simulink model "labA23"  (R2025b)
settings: Solver=ode45  StartTime=0.0  StopTime=300  RelTol=1e-3  AbsTol=1e-3  EnableMultiTasking=on
StopFcn:
  | %% Colors
  | 
  | blue = [0, 0.4470, 0.7410]; % RGB for blue
  | red = [0.8500, 0.3250, 0.0980]; % RGB for red
  | green = [0, 0.4980, 0]; % RGB for green
  | 
  | %% Data fetching
  | rt    = simout.u_v1.time; s.t=rt;  % time vector
  | ru_v1 = simout.u_v1.data; s.u_v1=ru_v1;
  | ru_v2 = simout.u_v2.data; s.u_v2=ru_v1;
  | ru_p  = simout.u_p.data;  s.u_p=ru_p;
  | rh1   = simout.measurement1.data; s.h1=rh1;
  | rh1_ref = simout.model1.data; s.h1_ref=rh1_ref;
  | rh2   = simout.measurement2.data; s.h2=rh2;
  | rh2_ref = simout.model2.data; s.h2_ref=rh2_ref;
  | 
  | %% Create figure
  | rslt = figure('Name','Results','Units','normalized', ...
  |               'Position',[0.25 0.2 0.5 0.5], ...
  |               'Color','w');
  | 
  | % Create tiled layout (3x2)
  | tl = tiledlayout(3,2,'Padding','compact','TileSpacing','compact');
  | 
  | %% Tile 1: u_v1
  | nexttile
  | plot(rt, ru_v1, 'Color', blue, 'LineWidth', 1.5)
  | xlabel('Time [s]')
  | ylabel('Valve signal u_{v1} [-]')
  | grid on;
  | 
  | %% Tile 2: h1
  | nexttile
  | plot(rt, rh1, 'Color', blue, 'LineWidth', 1.5)
  | hold on;
  | plot(rt, rh1_ref, 'Color', red, 'LineWidth', 1.5)
  | xlabel('Time [s]'); ylabel('Height h1 [m]'); grid on;
  | 
  | %% Tile 3: u_v2
  | nexttile
  | plot(rt, ru_v2, 'Color', blue, 'LineWidth', 1.5)
  | xlabel('Time [s]')
  | ylabel('Valve signal u_{v2} [-]')
  | grid on;
  | 
  | %% Tile 4: h2
  | nexttile
  | plot(rt, rh2, 'Color', blue, 'LineWidth', 1.5)
  | hold on;
  | plot(rt, rh2_ref, 'Color', red, 'LineWidth', 1.5)
  | xlabel('Time [s]'); ylabel('Height h2 [m]'); grid on;
  | 
  | %% Tile 5: u_p
  | nexttile
  | plot(rt, ru_p, 'Color', blue, 'LineWidth', 1.5)
  | xlabel('Time [s]')
  | ylabel('Pump signal u_{p} [-]')
  | grid on;
  | 
  | sgtitle('Results', 'FontWeight','bold');
undefined symbols (not defined in the file or in its folder): A1, f_v1, f_v2, g, h1_max, h1_min, h2_max, h2_min, h_v1, h_v2, k_v1, k_v2, q_p, rho, u_p, u_v1, u_v2, X, Y, Z
libraries: sm_lib x21, nesl_utility x8
settings Model: PacingRate=8  Creator=2922887  LastModifiedBy=danie
settings SolverCC: AutoScaleAbsTol=off  AlgebraicLoopSolver=TrustRegion
settings DataIOCC: LimitDataPoints=on  MaxDataPoints=10000  ReturnWorkspaceOutputs=off
settings OptimizationCC: LifeSpan=inf
settings DebuggingCC: UnconnectedInputMsg=warning  UnconnectedOutputMsg=warning  UnconnectedLineMsg=warning  AllowSymbolicDim=off  SFUnexpectedBacktrackingDiag=warning  SFNoUnconditionalDefaultTransitionDiag=warning  SFExecutionAtInitializationDiag=none  ArithmeticOperatorsInVariantConditions=warning
settings ModelReferenceCC: EnableRefExpFcnMdlSchedulingChecks=on
settings SFSimCC: SimUseLocalCustomCode=off  CustomCodeUndefinedFunction=UseInterfaceOnly
settings RTWCC: RTWUseLocalCustomCode=off  GPUComputeCapability=3.5  DLArmComputeVersion=19.05
settings CodeAppCC: StateflowObjectComments=on
settings GRTTargetCC: TargetLangStandard=C89/C90 (ANSI)
settings ConfigComp: CovMetricSettings=dw  CovSaveCumulativeToWorkspaceVar=on  CovSaveSingleToWorkspaceVar=on  CovExternalEMLEnable=off  CovSFcnEnable=off
settings SimscapeCC: SimscapeLogType=all  SimscapeLogSimulationStatistics=on  SimscapeLogDataHistory=10000.0
settings ExplorerConfigSet: InternalSimMechanicsExplorerSettings="<ExplorerConfiguration><canonicalview>default</canonicalview><AnimationSetting><BasePlaybackSpeed>1.0</BasePlaybackSpeed><PlaybackSpeedFactor>256.0</PlaybackSpeedFactor></AnimationSetting><TilePanel><TileInfo><Tiles Columns=\"1\" Count=\"1\" Rows=\"1\"><Column Weight=\"1\"/><Row Weight=\"1\"/><Tile Height=\"1\" Width=\"1\" X=\"0\" Y=\"0\"/></Tiles></TileInfo><SceneInfo><SceneViewer><BGColor><R>1</R><G>1</G><B>1</B></BGColor><Camera><DoPerspective>off</DoPerspective><Position><X>1.74662213976138903</X><Y>-0.732674940485340098</Y><Z>1.86695078489503663</Z></Position><Center><X>-0.869514407391283939</X><Y>0.382598842481733703</Y><Z>0.955734133281551657</Z></Center><Up><X>-0.285163512035032929</X><Y>0.109102028578263566</Y><Z>0.952249189426777054</Z></Up><ViewLimDist>1</ViewLimDist><YLim>1.42715679542026352</YLim><XLim>2.09465770497110215</XLim></Camera></SceneViewer></SceneInfo></TilePanel><MechEditorPanel><Cameras/><GfxPanelCameraMap/><VideoCreator><PlaybackSpeedRatio>1.0</PlaybackSpeedRatio><FrameRate>30</FrameRate><VideoFormat>Motion JPEG AVI</VideoFormat><FrameSize>auto</FrameSize></VideoCreator></MechEditorPanel></ExplorerConfiguration>"

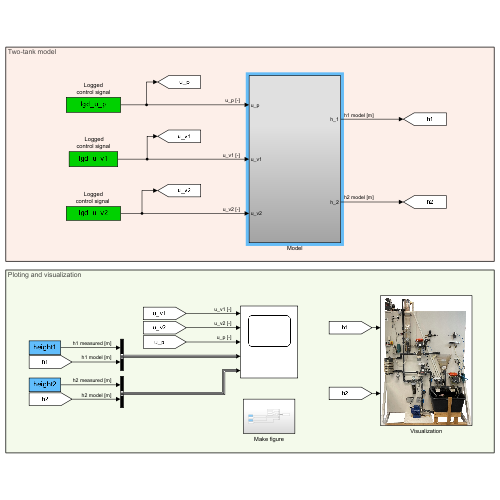
[thumbnail: Simulink's stored preview of the top-level diagram]
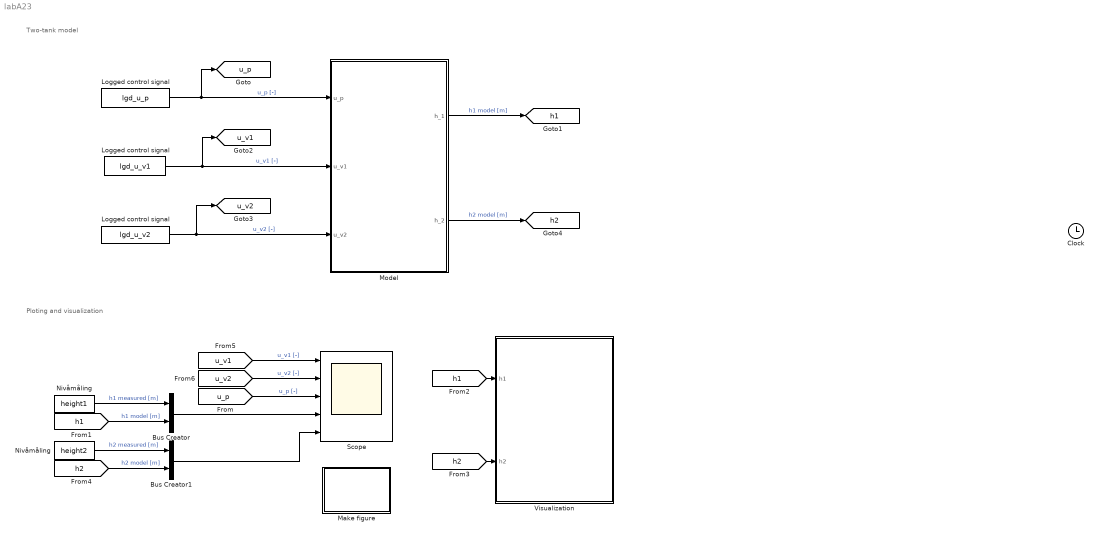
== system labA23 ==
  note: Ploting and visualization
  note: Two-tank model
  " Logged control signal" : FromWorkspace  VariableName=lgd_u_v1  SampleTime=0.07
  Bus Creator : BusCreator  Inputs=2
  Bus Creator1 : BusCreator  Inputs=2
  Logged control signal : FromWorkspace  VariableName=lgd_u_p  SampleTime=0.07
  "Logged control signal " : FromWorkspace  VariableName=lgd_u_v2  SampleTime=0.07
  Make figure : Subsystem
  Model : Subsystem
  Nivåmåling : FromWorkspace  VariableName=height1  SampleTime=0.07
  "Nivåmåling " : FromWorkspace  VariableName=height2  SampleTime=0.07
  Scope : Scope  NumInputPorts=5
      settings: TimeSpan=300  ActiveDisplayYMinimum=-0.125  ActiveDisplayYMaximum=1.125
  Visualization : Subsystem  mask{visualization=Visualization off, PacingRate=8}
      mask prompts: PacingRate "Simulation ratio (1:x) time vs real time"
      settings: PortSchema="{\"entries\":[{\"content\":{\"sides\":[{\"content\":{\"connectorIds\":[]},\"type\":\"ConnectorPlacement.EquallySpacedRectSide\",\"uuid\":\"ef884aaa-3eab-45c5-b5e8-52d600c009e8\"},{\"content\":{\"connectorIds\":[\"In1\",\"In2\"],\"side\":\"RIGHT\"},\"type\":\"ConnectorPlacement.EquallySpacedRectSide\",\"uuid\":\"bd48a19f-380a-480a-b360-7685a60cdefc\"},{\"content\":{\"connectorIds\":[],\"side\":\"TOP\"},\"type\":\"ConnectorPlacement.EquallySpacedRectSide\",\"uuid\":\"e0bb9c54-6b8d-425a-9dcd-efa9c2145964\"},{\"content\":{\"connectorIds\":[],\"side\":\"HIDDEN\"},\"type\":\"ConnectorPlacement.EquallySpacedRectSide\",\"uuid\":\"043d02d6-7b77-4bef-801d-231041ca0e56\"}]},\"type\":\"ConnectorPlacement.EquallySpacedConnector\",\"uuid\":\"8c6c52bd-5deb-48d7-b067-5e5f394c76bc\"}],\"packageUris\":[\"http://schema.mathworks.com/mf0/Connector/R2020b\"],\"version\":\"1.0\"}"
      mask TypeOptions visualization: Visualization  on | Visualization off
      mask Callback visualization:
      | if get_param(append(bdroot,'/Visualization'),'visualization') == 'Visualization  on'
      |    set_param(bdroot,'EnablePacing','on')
      | elseif get_param(append(bdroot,'/Visualization'),'visualization') == 'Visualization off'
      |    set_param(bdroot,'EnablePacing','off')
      | end
      mask Callback PacingRate:
      | temp_param = str2num(get_param(append(bdroot,'/Visualization'),'PacingRate'));
      | if temp_param >= 0.003 && temp_param < 0.0078
      |     set_param(bdroot,'PacingRate','0.0039')
      |     set_param(append(bdroot,'/Visualization'),'PacingRate','0.0039')
      | elseif temp_param >= 0.0078 && temp_param < 0.0156
      |     set_param(bdroot,'PacingRate','0.0078')
      |     set_param(append(bdroot,'/Visualization'),'PacingRate','0.0078')
      | elseif temp_param >= 0.0156 && temp_param < 0.0313
      |     set_param(bdroot,'PacingRate','0.0156')
      |     set_param(append(bdroot,'/Visualization'),'PacingRate','0.0156')
      | elseif temp_param >= 0.0313 && temp_param < 0.0625
      |     set_param(bdroot,'PacingRate','0.0313')
      |     set_param(append(bdroot,'/Visualization'),'PacingRate','0.0313')
      | elseif temp_param >= 0.0625 && temp_param < 0.1250
      |     set_param(bdroot,'PacingRate','0.0625')
      |     set_param(append(bdroot,'/Visualization'),'PacingRate','0.0625')
      | elseif temp_param >= 0.1250 && temp_param < 0.2500
      |     set_param(bdroot,'PacingRate','0.1250')
      |     set_param(append(bdroot,'/Visualization'),'PacingRate','0.1250')
      | elseif temp_param >= 0.2500 && temp_param < 0.5000
      |     set_param(bdroot, 'PacingRate','0.2500')
      |     set_param(append(bdroot,'/Visualization'),'PacingRate','0.2500')
      | elseif temp_param >= 0.5000 && temp_param < 1
      |     set_param(bdroot, 'PacingRate','0.5000')
      |     set_param(append(bdroot,'/Visualization'),'PacingRate','0.5000')
      | elseif temp_param >= 1 && temp_param < 2
      |     set_param(bdroot, 'PacingRate','1')
      |     set_param(append(bdroot,'/Visualization'),'PacingRate','1')
      | elseif temp_param >= 2 && temp_param < 4
      |     set_param(bdroot, 'PacingRate','2')
      |     set_param(append(bdroot,'/Visualization'),'PacingRate','2')
      | elseif temp_param >= 4 && temp_param < 8
      |     set_param(bdroot, 'PacingRate','4')
      |     set_param(append(bdroot,'/Visualization'),'PacingRate','4')
      | elseif temp_param >= 8 && temp_param < 16
      |     set_param(bdroot, 'PacingRate','8')
      |     set_param(append(bdroot,'/Visualization'),'PacingRate','8')
      | elseif temp_param >= 16 && temp_param < 32
      |     set_param(bdroot, 'PacingRate','16')
      |     set_param(append(bdroot,'/Visualization'),'PacingRate','16')
      | elseif temp_param >= 32 && temp_param < 64
      |     set_param(bdroot, 'PacingRate','32')
      |     set_param(append(bdroot,'/Visualization'),'PacingRate','32')
      | elseif temp_param >= 64 && temp_param < 128
      |     set_param(bdroot, 'PacingRate','64')
      |     set_param(append(bdroot,'/Visualization'),'PacingRate','64')
      | elseif temp_param >= 128 && temp_param < 256
      |     set_param(bdroot, 'PacingRate','128')
      |     set_param(append(bdroot,'/Visualisering'),'PacingRate','128')
      | elseif temp_param >= 256
      |     set_param(bdroot, 'PacingRate','256')
      |     set_param(append(bdroot,'/Visualization'),'PacingRate','256')
      | end
      mask DialogControl Control2 Prompt: For a 1:1 relation between the visualization model and the plotted data, the simulation ratio in this box should match the ratio in the Mechanics Explorer.
      mask DialogControl x256x Prompt: 0.0039 = 1/256x
      mask DialogControl x128x Prompt: 0.0078 = 1/128x
      mask DialogControl x64x Prompt: 0.0156 = 1/64x
      mask DialogControl x32x Prompt: 0.0313 = 1/32x
      mask DialogControl x16x Prompt: 0.0625 = 1/16x
      mask DialogControl x8x Prompt: 0.1250 = 1/8x
      mask DialogControl x4x Prompt: 0.2500 = 1/4x
      mask DialogControl x2x Prompt: 0.5000 = 1/2x
      mask Display: image('$imagefile'); % Use "Edit Image" on toolstrip to change.
  Clock : Clock
      settings: IOType=siggen
  tag scope: h1=global, h2=global, u_p=global, u_v1=global, u_v2=global
  wires:
  " Logged control signal"/1 -> [u_v1], Model/2(u_v1)  "u_v1 [-]"
  Model/1(h_1) -> [h1]  "h1 model [m]"
  Logged control signal/1 -> [u_p], Model/1(u_p)  "u_p [-]"
  Nivåmåling/1 -> Bus Creator/1  "h1 measured [m]"
  "Logged control signal "/1 -> [u_v2], Model/3(u_v2)  "u_v2 [-]"
  Model/2(h_2) -> [h2]  "h2 model [m]"
  [h1] -> Visualization/1(h1)
  [h2] -> Visualization/2(h2)
  [h1] -> Bus Creator/2  "h1 model [m]"
  [h2] -> Bus Creator1/2  "h2 model [m]"
  "Nivåmåling "/1 -> Bus Creator1/1  "h2 measured [m]"
  Bus Creator1/1 -> Scope/5
  Bus Creator/1 -> Scope/4
  [u_v2] -> Scope/2  "u_v2 [-]"
  [u_v1] -> Scope/1  "u_v1 [-]"
  [u_p] -> Scope/3  "u_p [-]"

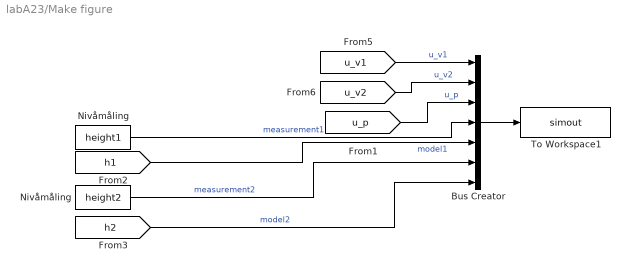
== system labA23/Make figure ==
  Bus Creator : BusCreator  Inputs=7
  Nivåmåling : FromWorkspace  VariableName=height1  SampleTime=0.07
  "Nivåmåling " : FromWorkspace  VariableName=height2  SampleTime=0.07
  To Workspace1 : ToWorkspace  VariableName=simout  SaveFormat=Timeseries  SampleTime=0.07
  wires:
  Bus Creator/1 -> To Workspace1/1
  [u_v1] -> Bus Creator/1  "u_v1"
  [u_v2] -> Bus Creator/2  "u_v2"
  [u_p] -> Bus Creator/3  "u_p"
  Nivåmåling/1 -> Bus Creator/4  "measurement1"
  [h1] -> Bus Creator/5  "model1"
  "Nivåmåling "/1 -> Bus Creator/6  "measurement2"
  [h2] -> Bus Creator/7  "model2"

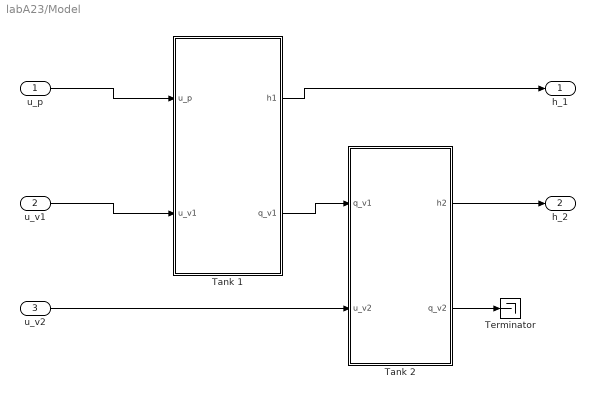
== system labA23/Model ==
  u_p : Inport
  u_v1 : Inport  Port=2
  u_v2 : Inport  Port=3
  Tank 1 : Subsystem
  Tank 2 : Subsystem
  Terminator : Terminator
  h_1 : Outport  VectorParamsAs1DForOutWhenUnconnected=off
  h_2 : Outport  Port=2  VectorParamsAs1DForOutWhenUnconnected=off
  wires:
  u_v1/1 -> Tank 1/2(u_v1)
  u_p/1 -> Tank 1/1(u_p)
  Tank 1/1(h1) -> h_1/1
  Tank 1/2(q_v1) -> Tank 2/1(q_v1)
  Tank 2/1(h2) -> h_2/1
  u_v2/1 -> Tank 2/2(u_v2)
  Tank 2/2(q_v2) -> Terminator/1

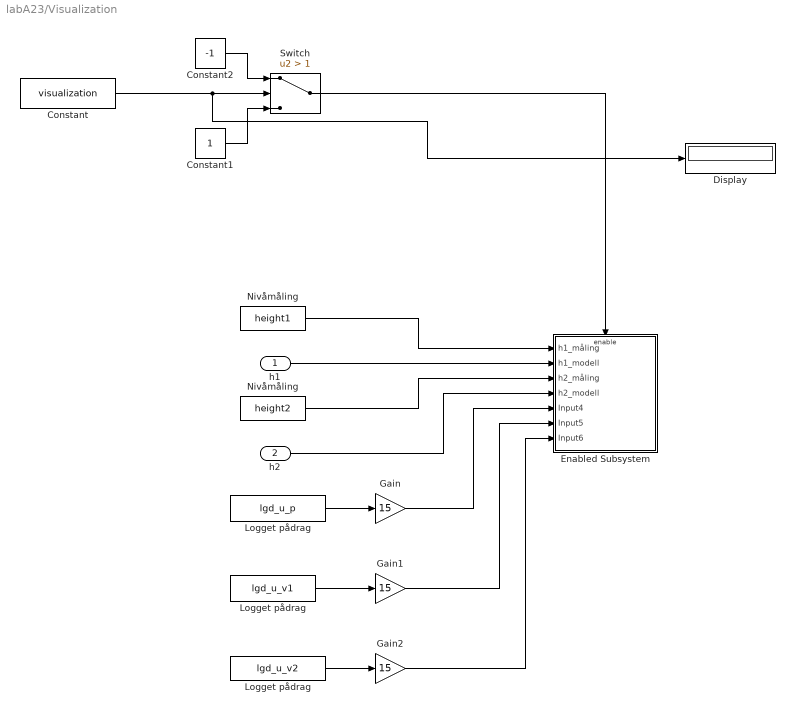
== system labA23/Visualization ==
  h1 : Inport
  h2 : Inport  Port=2
  Constant : Constant  Value=visualization
  Constant1 : Constant
  Constant2 : Constant  Value=-1
  Display : Display
  Enabled Subsystem : Subsystem  TreatAsAtomicUnit=on
  Gain : Gain  Gain=15
  Gain1 : Gain  Gain=15
  Gain2 : Gain  Gain=15
  Logget pådrag : FromWorkspace  VariableName=lgd_u_p  SampleTime=0.07
  "Logget pådrag " : FromWorkspace  VariableName=lgd_u_v1  SampleTime=0.07
  "Logget pådrag  " : FromWorkspace  VariableName=lgd_u_v2  SampleTime=0.07
  Nivåmåling : FromWorkspace  VariableName=height1  SampleTime=0.07
  "Nivåmåling " : FromWorkspace  VariableName=height2  SampleTime=0.07
  Switch : Switch  Criteria=u2 > Threshold  Threshold=1  SaturateOnIntegerOverflow=off  InputSameDT=off
  wires:
  Constant1/1 -> Switch/3
  Constant2/1 -> Switch/1
  Switch/1 -> Enabled Subsystem/Enable
  Constant/1 -> Display/1, Switch/2
  "Nivåmåling "/1 -> Enabled Subsystem/3(h2_måling)
  Nivåmåling/1 -> Enabled Subsystem/1(h1_måling)
  "Logget pådrag "/1 -> Gain1/1
  "Logget pådrag  "/1 -> Gain2/1
  Logget pådrag/1 -> Gain/1
  Gain/1 -> Enabled Subsystem/5(Input4)
  Gain1/1 -> Enabled Subsystem/6(Input5)
  Gain2/1 -> Enabled Subsystem/7(Input6)
  h1/1 -> Enabled Subsystem/2(h1_modell)
  h2/1 -> Enabled Subsystem/4(h2_modell)

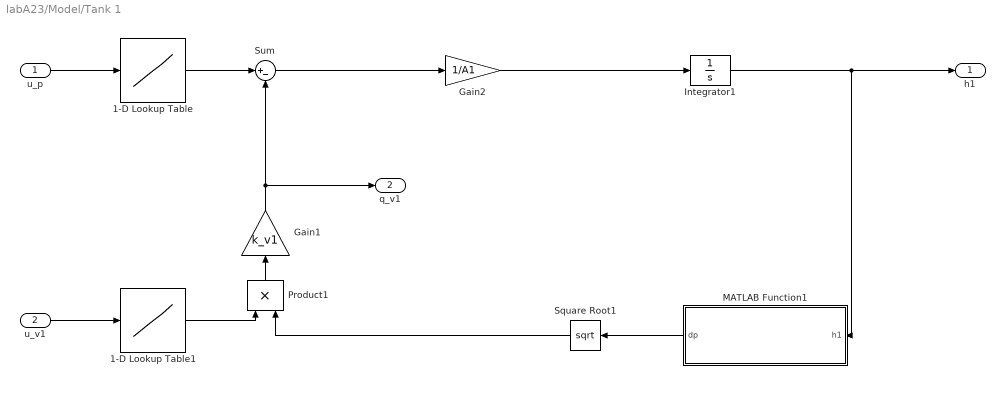
== system labA23/Model/Tank 1 ==
  u_p : Inport
  u_v1 : Inport  Port=2
  1-D Lookup Table : Lookup_n-D  NumberOfTableDimensions=1  BreakpointsForDimension1=u_p  Table=q_p  InternalRulePriority=Speed  RndMeth=Simplest
  1-D Lookup Table1 : Lookup_n-D  NumberOfTableDimensions=1  BreakpointsForDimension1=u_v1  Table=f_v1  InternalRulePriority=Speed  RndMeth=Simplest
  Gain1 : Gain  Gain=k_v1
  Gain2 : Gain  Gain=1/A1
  Integrator1 : Integrator  InitialCondition=h1_min  LimitOutput=on  UpperSaturationLimit=h1_max  LowerSaturationLimit=h1_min
  MATLAB Function1 : MATLAB Function  TreatAsAtomicUnit=on
  Product1 : Product
  Square Root1 : Sqrt
  Sum : Sum  Inputs=|+-
  h1 : Outport
  q_v1 : Outport  Port=2
  wires:
  u_p/1 -> 1-D Lookup Table/1
  Square Root1/1 -> Product1/2
  Gain2/1 -> Integrator1/1
  Sum/1 -> Gain2/1
  u_v1/1 -> 1-D Lookup Table1/1
  Integrator1/1 -> MATLAB Function1/1(h1), h1/1
  1-D Lookup Table1/1 -> Product1/1
  1-D Lookup Table/1 -> Sum/1
  Product1/1 -> Gain1/1
  MATLAB Function1/1(dp) -> Square Root1/1
  Gain1/1 -> Sum/2, q_v1/1

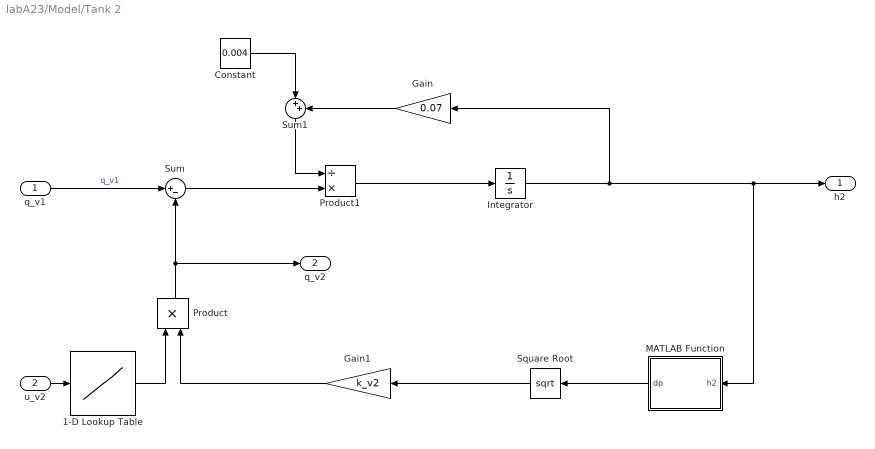
== system labA23/Model/Tank 2 ==
  q_v1 : Inport
  u_v2 : Inport  Port=2
  1-D Lookup Table : Lookup_n-D  NumberOfTableDimensions=1  BreakpointsForDimension1=u_v2  Table=f_v2  InternalRulePriority=Speed  RndMeth=Simplest
  Constant : Constant  Value=0.004
  Gain : Gain  Gain=0.07
  Gain1 : Gain  Gain=k_v2
  Integrator : Integrator  InitialCondition=h2_min  LimitOutput=on  UpperSaturationLimit=h2_max  LowerSaturationLimit=h2_min
  MATLAB Function : MATLAB Function  TreatAsAtomicUnit=on
  Product : Product
  Product1 : Product  Inputs=/*
  Square Root : Sqrt
  Sum : Sum  Inputs=|+-
  Sum1 : Sum  Inputs=|++
  h2 : Outport  VectorParamsAs1DForOutWhenUnconnected=off
  q_v2 : Outport  Port=2  VectorParamsAs1DForOutWhenUnconnected=off
  wires:
  u_v2/1 -> 1-D Lookup Table/1
  Product/1 -> q_v2/1, Sum/2
  q_v1/1 -> Sum/1  "q_v1"
  Integrator/1 -> MATLAB Function/1(h2), h2/1, Gain/1
  Gain/1 -> Sum1/2
  Constant/1 -> Sum1/1
  Sum/1 -> Product1/2
  Sum1/1 -> Product1/1
  Gain1/1 -> Product/2
  1-D Lookup Table/1 -> Product/1
  Square Root/1 -> Gain1/1
  MATLAB Function/1(dp) -> Square Root/1
  Product1/1 -> Integrator/1

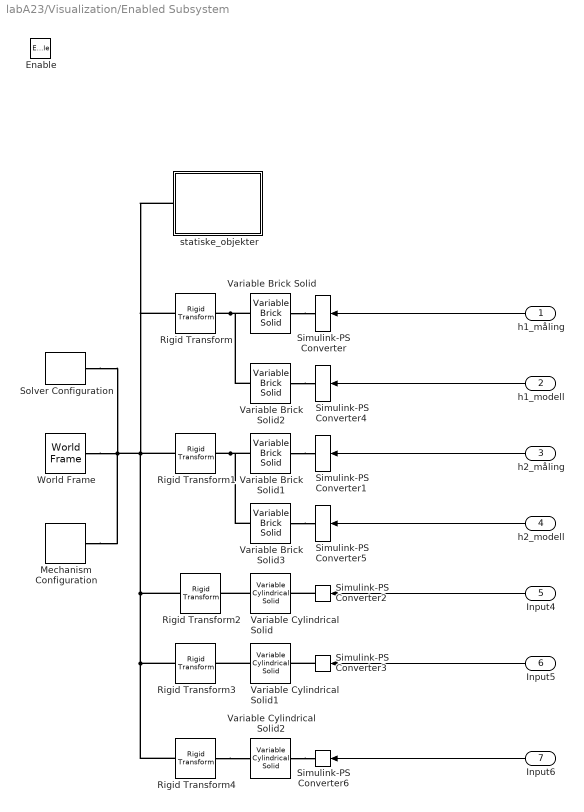
== system labA23/Visualization/Enabled Subsystem ==
  h1_måling : Inport
  h1_modell : Inport  Port=2
  h2_måling : Inport  Port=3
  h2_modell : Inport  Port=4
  Input4 : Inport  Port=5
  Input5 : Inport  Port=6
  Input6 : Inport  Port=7
  Enable : EnablePort
  Mechanism Configuration : sm_lib/Utilities/Mechanism Configuration  UniformGravity=Constant  GravityVector=[0 0 -9.80665]  GravityVectorUnits=m/s^2  LinearizationDelta=0.001  JointModeTransitionNonlinearIterations=2
  Rigid Transform : sm_lib/Frames and Transforms/Rigid Transform  RotationMethod=None  FollAlignAxisA=+X  BaseAlignAxisA=+Y  FollAlignAxisB=+Y  BaseAlignAxisB=+Z  RotationStandardAxis=+Z  RotationAngle=0.0  RotationAngleUnits=deg  RotationArbitraryAxis=[0 0 1]  RotationSequenceAxes=FollowerAxes  RotationSequence=XYX  RotationSequenceAngles=[0 0 0]  RotationSequenceAnglesUnits=deg  RotationMatrix=[1 0 0; 0 1 0; 0 0 1]  Quaternion=[1 0 0 0]  TranslationMethod=Cartesian  TranslationCartesianOffset=[46 -468 1498]  TranslationCartesianOffsetUnits=mm  TranslationStandardAxis=+Z  TranslationStandardOffset=0  TranslationStandardOffsetUnits=mm  TranslationROffset=0  TranslationROffsetUnits=m  TranslationThetaOffset=0  TranslationThetaOffsetUnits=deg  TranslationZOffset=0  TranslationZOffsetUnits=m
  Rigid Transform1 : sm_lib/Frames and Transforms/Rigid Transform  RotationMethod=None  FollAlignAxisA=+X  BaseAlignAxisA=+Y  FollAlignAxisB=+Y  BaseAlignAxisB=+Z  RotationStandardAxis=+Z  RotationAngle=0.0  RotationAngleUnits=deg  RotationArbitraryAxis=[0 0 1]  RotationSequenceAxes=FollowerAxes  RotationSequence=XYX  RotationSequenceAngles=[0 0 0]  RotationSequenceAnglesUnits=deg  RotationMatrix=[1 0 0; 0 1 0; 0 0 1]  Quaternion=[1 0 0 0]  TranslationMethod=Cartesian  TranslationCartesianOffset=[46 530 978]  TranslationCartesianOffsetUnits=mm  TranslationStandardAxis=+Z  TranslationStandardOffset=0  TranslationStandardOffsetUnits=mm  TranslationROffset=0  TranslationROffsetUnits=m  TranslationThetaOffset=0  TranslationThetaOffsetUnits=deg  TranslationZOffset=0  TranslationZOffsetUnits=m
  Rigid Transform2 : sm_lib/Frames and Transforms/Rigid Transform  RotationMethod=None  FollAlignAxisA=+X  BaseAlignAxisA=+Y  FollAlignAxisB=+Y  BaseAlignAxisB=+Z  RotationStandardAxis=+Z  RotationAngle=0.0  RotationAngleUnits=deg  RotationArbitraryAxis=[0 0 1]  RotationSequenceAxes=FollowerAxes  RotationSequence=XYX  RotationSequenceAngles=[0 0 0]  RotationSequenceAnglesUnits=deg  RotationMatrix=[1 0 0; 0 1 0; 0 0 1]  Quaternion=[1 0 0 0]  TranslationMethod=Cartesian  TranslationCartesianOffset=[46 -500 1498]  TranslationCartesianOffsetUnits=mm  TranslationStandardAxis=+Z  TranslationStandardOffset=0  TranslationStandardOffsetUnits=mm  TranslationROffset=0  TranslationROffsetUnits=m  TranslationThetaOffset=0  TranslationThetaOffsetUnits=deg  TranslationZOffset=0  TranslationZOffsetUnits=m
  Rigid Transform3 : sm_lib/Frames and Transforms/Rigid Transform  RotationMethod=None  FollAlignAxisA=+X  BaseAlignAxisA=+Y  FollAlignAxisB=+Y  BaseAlignAxisB=+Z  RotationStandardAxis=+Z  RotationAngle=0.0  RotationAngleUnits=deg  RotationArbitraryAxis=[0 0 1]  RotationSequenceAxes=FollowerAxes  RotationSequence=XYX  RotationSequenceAngles=[0 0 0]  RotationSequenceAnglesUnits=deg  RotationMatrix=[1 0 0; 0 1 0; 0 0 1]  Quaternion=[1 0 0 0]  TranslationMethod=Cartesian  TranslationCartesianOffset=[46 500.698 978]  TranslationCartesianOffsetUnits=mm  TranslationStandardAxis=+Z  TranslationStandardOffset=0  TranslationStandardOffsetUnits=mm  TranslationROffset=0  TranslationROffsetUnits=m  TranslationThetaOffset=0  TranslationThetaOffsetUnits=deg  TranslationZOffset=0  TranslationZOffsetUnits=m
  Rigid Transform4 : sm_lib/Frames and Transforms/Rigid Transform  RotationMethod=RotationSequence  FollAlignAxisA=+X  BaseAlignAxisA=+Y  FollAlignAxisB=+Y  BaseAlignAxisB=+Z  RotationStandardAxis=+Z  RotationAngle=0.0  RotationAngleUnits=deg  RotationArbitraryAxis=[0 0 1]  RotationSequenceAxes=FollowerAxes  RotationSequence=XYX  RotationSequenceAngles=[136.1 15 0]  RotationSequenceAnglesUnits=deg  RotationMatrix=[1 0 0; 0 1 0; 0 0 1]  Quaternion=[1 0 0 0]  TranslationMethod=Cartesian  TranslationCartesianOffset=[212.728 726.645 608.857]  TranslationCartesianOffsetUnits=mm  TranslationStandardAxis=+Z  TranslationStandardOffset=0  TranslationStandardOffsetUnits=mm  TranslationROffset=0  TranslationROffsetUnits=m  TranslationThetaOffset=0  TranslationThetaOffsetUnits=deg  TranslationZOffset=0  TranslationZOffsetUnits=m
  Simulink-PS Converter{,1,4..5} (4 alike) : nesl_utility/Simulink-PS Converter  PhysicalDomain=network_engine_domain  SubClassName=ps_input  LeftPortType=input  RightPortType=output  PseudoPeriodic=off  Frequencies=[]  NoiseDistribution=none  NoiseParameters=[]  Unit=m  AffineConversion=off  FilteringAndDerivatives=filter  SimscapeFilterOrder=2  InputFilterTimeConstant=0.01  UdotUserProvided=0
  Simulink-PS Converter2 : nesl_utility/Simulink-PS Converter  PhysicalDomain=network_engine_domain  SubClassName=ps_input  LeftPortType=input  RightPortType=output  PseudoPeriodic=off  Frequencies=[]  NoiseDistribution=none  NoiseParameters=[]  Unit=mm  AffineConversion=off  FilteringAndDerivatives=filter  SimscapeFilterOrder=2  InputFilterTimeConstant=0.01  UdotUserProvided=0
  Simulink-PS Converter3 : nesl_utility/Simulink-PS Converter  PhysicalDomain=network_engine_domain  SubClassName=ps_input  LeftPortType=input  RightPortType=output  PseudoPeriodic=off  Frequencies=[]  NoiseDistribution=none  NoiseParameters=[]  Unit=mm  AffineConversion=off  FilteringAndDerivatives=filter  SimscapeFilterOrder=2  InputFilterTimeConstant=0.01  UdotUserProvided=0
  Simulink-PS Converter6 : nesl_utility/Simulink-PS Converter  PhysicalDomain=network_engine_domain  SubClassName=ps_input  LeftPortType=input  RightPortType=output  PseudoPeriodic=off  Frequencies=[]  NoiseDistribution=none  NoiseParameters=[]  Unit=mm  AffineConversion=off  FilteringAndDerivatives=filter  SimscapeFilterOrder=2  InputFilterTimeConstant=0.01  UdotUserProvided=0
  Solver Configuration : nesl_utility/Solver Configuration  PhysicalDomain=network_engine_domain  SubClassName=solver  LeftPortType=input  RightPortType=generic  Tones=[]  Harmonics=[]  SimulateNoise=off  Profile=off  UseLocalSampling=off  EnableSwitchedLinearOptims=on  FrequencyDomain=off  UseCCode=off  RelTol=0.001  AbsTol=1e-06  MinStep=1e-09  ToWorkspace=off  RevertToSquareIcSolve=off  NumHomotopyIterations=100  PhasorMode=off  PhasorModeNumHarmonics=1  ConsistencySolver=NEWTON_FTOL  IndexReductionMethod=DerivativeReplacement  DoDC=off  ResidualTolerance=1e-09  ConsistencyTolSource=GLOBAL  ConsistencyAbsTol=0.001  ConsistencyRelTol=0.001  ConsistencyTolFactor=0.001  UseLocalSolver=off  LocalSolverChoice=NE_BACKWARD_EULER_ADVANCER  ResolveIndetEquations=on  FunctionEvalNumThread=1  LocalSolverSampleTime=0.001  DoFixedCost=off  MaxNonlinIter=3  MaxModeIter=2  ComputeImpulses=off  ImpulseIterations=2  LinearAlgebra=Sparse  LinearAlgebraNumThread=0  EquationFormulation=NE_TIME_EF  DelaysMemoryBudget=1024  AutomaticFiltering=on  FilteringTimeConstant=0.001  PartitionStorageMethod=AS_NEEDED  PartitionMemoryBudget=1024  PartitionMethod=FAST  MultibodyUseLocalSolver=off  MultibodyLocalSolverChoice=ODE1  MultibodyLocalSolverSampleTime=0.001
  Variable Brick Solid : sm_lib/Body Elements/Variable Mass/Variable Brick Solid  XLengthType=Constant  XLength=80  XLengthUnits=mm  YLengthType=Constant  YLength=123  YLengthUnits=mm  ZLengthType=ProvidedByInput  ZLength=1  ZLengthUnits=m  MassType=CalculateFromGeometry  Density=1000  DensityUnits=kg/m^3  SenseXLength=off  SenseYLength=off  SenseZLength=off  SenseMass=off  SenseCenterOfMass=off  SenseInertiaMatrix=off  GraphicType=FromGeometry  MarkerShape=Sphere  MarkerSize=10  GraphicVisPropType=SimpleVisualProperties  GraphicDiffuseColor=[0.4 0.8 1.0]  GraphicOpacity=0.8  GraphicSpecularColor=[0.5 0.5 0.5 1.0]  GraphicAmbientColor=[0.15 0.15 0.15 1.0]  GraphicEmissiveColor=[0.0 0.0 0.0 1.0]  GraphicShininess=75
  Variable Brick Solid1 : sm_lib/Body Elements/Variable Mass/Variable Brick Solid  XLengthType=Constant  XLength=79  XLengthUnits=mm  YLengthType=Constant  YLength=410  YLengthUnits=mm  ZLengthType=ProvidedByInput  ZLength=1  ZLengthUnits=m  MassType=CalculateFromGeometry  Density=1000  DensityUnits=kg/m^3  SenseXLength=off  SenseYLength=off  SenseZLength=off  SenseMass=off  SenseCenterOfMass=off  SenseInertiaMatrix=off  GraphicType=FromGeometry  MarkerShape=Sphere  MarkerSize=100  GraphicVisPropType=AdvancedVisualProperties  GraphicDiffuseColor=[0.4 0.8 1.0]  GraphicOpacity=0.8  GraphicSpecularColor=[0.5 0.5 0.5 1.0]  GraphicAmbientColor=[0.15 0.15 0.15 1.0]  GraphicEmissiveColor=[0.0 0.0 0.0 1.0]  GraphicShininess=75
  Variable Brick Solid2 : sm_lib/Body Elements/Variable Mass/Variable Brick Solid  XLengthType=Constant  XLength=78  XLengthUnits=mm  YLengthType=Constant  YLength=122  YLengthUnits=mm  ZLengthType=ProvidedByInput  ZLength=1  ZLengthUnits=m  MassType=CalculateFromGeometry  Density=1000  DensityUnits=kg/m^3  SenseXLength=off  SenseYLength=off  SenseZLength=off  SenseMass=off  SenseCenterOfMass=off  SenseInertiaMatrix=off  GraphicType=FromGeometry  MarkerShape=Sphere  MarkerSize=10  GraphicVisPropType=SimpleVisualProperties  GraphicDiffuseColor=[0.0 0.2 1.0]  GraphicOpacity=1  GraphicSpecularColor=[0.5 0.5 0.5 1.0]  GraphicAmbientColor=[0.15 0.15 0.15 1.0]  GraphicEmissiveColor=[0.0 0.0 0.0 1.0]  GraphicShininess=75
  Variable Brick Solid3 : sm_lib/Body Elements/Variable Mass/Variable Brick Solid  XLengthType=Constant  XLength=77  XLengthUnits=mm  YLengthType=Constant  YLength=410  YLengthUnits=mm  ZLengthType=ProvidedByInput  ZLength=1  ZLengthUnits=m  MassType=CalculateFromGeometry  Density=1000  DensityUnits=kg/m^3  SenseXLength=off  SenseYLength=off  SenseZLength=off  SenseMass=off  SenseCenterOfMass=off  SenseInertiaMatrix=off  GraphicType=FromGeometry  MarkerShape=Sphere  MarkerSize=10  GraphicVisPropType=SimpleVisualProperties  GraphicDiffuseColor=[0.0 0.2 1.0]  GraphicOpacity=1  GraphicSpecularColor=[0.5 0.5 0.5 1.0]  GraphicAmbientColor=[0.15 0.15 0.15 1.0]  GraphicEmissiveColor=[0.0 0.0 0.0 1.0]  GraphicShininess=75
  Variable Cylindrical Solid : sm_lib/Body Elements/Variable Mass/Variable Cylindrical Solid  RadiusType=ProvidedByInput  Radius=1  RadiusUnits=m  LengthType=Constant  Length=965  LengthUnits=mm  MassType=CalculateFromGeometry  Density=1000  DensityUnits=kg/m^3  SenseRadius=off  SenseLength=off  SenseMass=off  SenseCenterOfMass=off  SenseInertiaMatrix=off  GraphicType=FromGeometry  MarkerShape=Sphere  MarkerSize=10  GraphicVisPropType=SimpleVisualProperties  GraphicDiffuseColor=[0.4 0.8 1.0]  GraphicOpacity=0.8  GraphicSpecularColor=[0.5 0.5 0.5 1.0]  GraphicAmbientColor=[0.15 0.15 0.15 1.0]  GraphicEmissiveColor=[0.0 0.0 0.0 1.0]  GraphicShininess=75
  Variable Cylindrical Solid1 : sm_lib/Body Elements/Variable Mass/Variable Cylindrical Solid  RadiusType=ProvidedByInput  Radius=1  RadiusUnits=m  LengthType=Constant  Length=395  LengthUnits=mm  MassType=CalculateFromGeometry  Density=1000  DensityUnits=kg/m^3  SenseRadius=off  SenseLength=off  SenseMass=off  SenseCenterOfMass=off  SenseInertiaMatrix=off  GraphicType=FromGeometry  MarkerShape=Sphere  MarkerSize=10  GraphicVisPropType=SimpleVisualProperties  GraphicDiffuseColor=[0.4 0.8 1.0]  GraphicOpacity=0.8  GraphicSpecularColor=[0.5 0.5 0.5 1.0]  GraphicAmbientColor=[0.15 0.15 0.15 1.0]  GraphicEmissiveColor=[0.0 0.0 0.0 1.0]  GraphicShininess=75
  Variable Cylindrical Solid2 : sm_lib/Body Elements/Variable Mass/Variable Cylindrical Solid  RadiusType=ProvidedByInput  Radius=15  RadiusUnits=mm  LengthType=Constant  Length=330  LengthUnits=mm  MassType=CalculateFromGeometry  Density=1000  DensityUnits=kg/m^3  SenseRadius=off  SenseLength=off  SenseMass=off  SenseCenterOfMass=off  SenseInertiaMatrix=off  GraphicType=FromGeometry  MarkerShape=Sphere  MarkerSize=10  GraphicVisPropType=SimpleVisualProperties  GraphicDiffuseColor=[0.4 0.8 1.0]  GraphicOpacity=0.8  GraphicSpecularColor=[0.5 0.5 0.5 1.0]  GraphicAmbientColor=[0.15 0.15 0.15 1.0]  GraphicEmissiveColor=[0.0 0.0 0.0 1.0]  GraphicShininess=75
  World Frame : sm_lib/Frames and Transforms/World Frame
  statiske_objekter : Subsystem
  wires:
  Input6/1 -> Simulink-PS Converter6/1
  Input5/1 -> Simulink-PS Converter3/1
  Input4/1 -> Simulink-PS Converter2/1
  h2_modell/1 -> Simulink-PS Converter5/1
  h2_måling/1 -> Simulink-PS Converter1/1
  h1_modell/1 -> Simulink-PS Converter4/1
  h1_måling/1 -> Simulink-PS Converter/1
  connections:
  Rigid Transform1/RConn1 -- Variable Brick Solid1/RConn1 -- Variable Brick Solid3/RConn1
  Rigid Transform3/LConn1 -- Mechanism Configuration/RConn1 -- World Frame/RConn1 -- Solver Configuration/RConn1 -- statiske_objekter/LConn1 -- Rigid Transform/LConn1 -- Rigid Transform1/LConn1 -- Rigid Transform2/LConn1 -- Rigid Transform4/LConn1
  Rigid Transform/RConn1 -- Variable Brick Solid/RConn1 -- Variable Brick Solid2/RConn1
  Variable Brick Solid2/LConn1 -- Simulink-PS Converter4/RConn1
  Variable Brick Solid1/LConn1 -- Simulink-PS Converter1/RConn1
  Variable Brick Solid3/LConn1 -- Simulink-PS Converter5/RConn1
  Simulink-PS Converter2/RConn1 -- Variable Cylindrical Solid/LConn1
  Variable Cylindrical Solid/RConn1 -- Rigid Transform2/RConn1
  Variable Brick Solid/LConn1 -- Simulink-PS Converter/RConn1
  Rigid Transform4/RConn1 -- Variable Cylindrical Solid2/RConn1
  Variable Cylindrical Solid2/LConn1 -- Simulink-PS Converter6/RConn1
  Simulink-PS Converter3/RConn1 -- Variable Cylindrical Solid1/LConn1
  Variable Cylindrical Solid1/RConn1 -- Rigid Transform3/RConn1

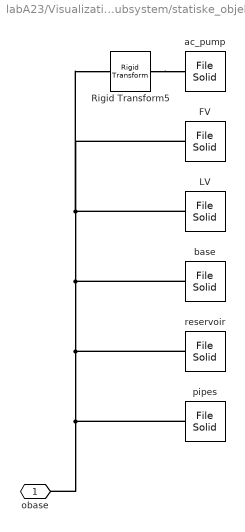
== system labA23/Visualization/Enabled Subsystem/statiske_objekter ==
  FV : sm_lib/Body Elements/File Solid  ExtGeomFileName=fv.stl  UnitType=Custom  ExtGeomFileUnits=mm  StepReaderType=HEX  ExportConvexHullGeometry=off  InertiaType=Custom  BasedOnType=DensityFromFile  Density=1000  DensityUnits=kg/m^3  Mass=1  MassUnits=kg  CenterOfMass=[0 0 0]  CenterOfMassUnits=m  MomentsOfInertia=[1 1 1]  MomentsOfInertiaUnits=kg*m^2  ProductsOfInertia=[0 0 0]  ProductsOfInertiaUnits=kg*m^2  GraphicType=FromGeometry  MarkerShape=Sphere  MarkerSize=10  GraphicVisPropType=SimpleVisualProperties  GraphicDiffuseColor=[1.0 0.6 0.0]  GraphicOpacity=1  GraphicSpecularColor=[0.5 0.5 0.5 1.0]  GraphicAmbientColor=[0.15 0.15 0.15 1.0]  GraphicEmissiveColor=[0.0 0.0 0.0 1.0]  GraphicShininess=75  DoExposeReferenceFrame=on  SerializedFrames=<Frames/>
  LV : sm_lib/Body Elements/File Solid  ExtGeomFileName=lv.stl  UnitType=Custom  ExtGeomFileUnits=mm  StepReaderType=HEX  ExportConvexHullGeometry=off  InertiaType=Custom  BasedOnType=DensityFromFile  Density=1000  DensityUnits=kg/m^3  Mass=1  MassUnits=kg  CenterOfMass=[0 0 0]  CenterOfMassUnits=m  MomentsOfInertia=[1 1 1]  MomentsOfInertiaUnits=kg*m^2  ProductsOfInertia=[0 0 0]  ProductsOfInertiaUnits=kg*m^2  GraphicType=FromGeometry  MarkerShape=Sphere  MarkerSize=10  GraphicVisPropType=SimpleVisualProperties  GraphicDiffuseColor=[1.0 0.0 0.0]  GraphicOpacity=1  GraphicSpecularColor=[0.5 0.5 0.5 1.0]  GraphicAmbientColor=[0.15 0.15 0.15 1.0]  GraphicEmissiveColor=[0.0 0.0 0.0 1.0]  GraphicShininess=75  DoExposeReferenceFrame=on  SerializedFrames=<Frames/>
  Rigid Transform5 : sm_lib/Frames and Transforms/Rigid Transform  RotationMethod=RotationSequence  FollAlignAxisA=+X  BaseAlignAxisA=+Y  FollAlignAxisB=+Y  BaseAlignAxisB=+Z  RotationStandardAxis=+Z  RotationAngle=0.0  RotationAngleUnits=deg  RotationArbitraryAxis=[0 0 1]  RotationSequenceAxes=FollowerAxes  RotationSequence=XYZ  RotationSequenceAngles=[90 180 0]  RotationSequenceAnglesUnits=deg  RotationMatrix=[1 0 0; 0 1 0; 0 0 1]  Quaternion=[1 0 0 0]  TranslationMethod=Cartesian  TranslationCartesianOffset=[107.68 -50.5 194]  TranslationCartesianOffsetUnits=mm  TranslationStandardAxis=+Z  TranslationStandardOffset=0  TranslationStandardOffsetUnits=mm  TranslationROffset=0  TranslationROffsetUnits=m  TranslationThetaOffset=0  TranslationThetaOffsetUnits=deg  TranslationZOffset=0  TranslationZOffsetUnits=m
  ac_pump : sm_lib/Body Elements/File Solid  ExtGeomFileName=pump.stl  UnitType=Custom  ExtGeomFileUnits=mm  StepReaderType=HEX  ExportConvexHullGeometry=off  InertiaType=Custom  BasedOnType=DensityFromFile  Density=1000  DensityUnits=kg/m^3  Mass=1  MassUnits=kg  CenterOfMass=[0 0 0]  CenterOfMassUnits=m  MomentsOfInertia=[1 1 1]  MomentsOfInertiaUnits=kg*m^2  ProductsOfInertia=[0 0 0]  ProductsOfInertiaUnits=kg*m^2  GraphicType=FromGeometry  MarkerShape=Sphere  MarkerSize=10  GraphicVisPropType=SimpleVisualProperties  GraphicDiffuseColor=[0.0 0.0 1.0]  GraphicOpacity=1  GraphicSpecularColor=[0.5 0.5 0.5 1.0]  GraphicAmbientColor=[0.15 0.15 0.15 1.0]  GraphicEmissiveColor=[0.0 0.0 0.0 1.0]  GraphicShininess=75  DoExposeReferenceFrame=on  SerializedFrames=<Frames/>
  base : sm_lib/Body Elements/File Solid  ExtGeomFileName=base.stl  UnitType=Custom  ExtGeomFileUnits=mm  StepReaderType=HEX  ExportConvexHullGeometry=off  InertiaType=Custom  BasedOnType=DensityFromFile  Density=1000  DensityUnits=kg/m^3  Mass=1  MassUnits=kg  CenterOfMass=[0 0 0]  CenterOfMassUnits=m  MomentsOfInertia=[1 1 1]  MomentsOfInertiaUnits=kg*m^2  ProductsOfInertia=[0 0 0]  ProductsOfInertiaUnits=kg*m^2  GraphicType=FromGeometry  MarkerShape=Sphere  MarkerSize=10  GraphicVisPropType=SimpleVisualProperties  GraphicDiffuseColor=[1.0 1.0 1.0]  GraphicOpacity=1  GraphicSpecularColor=[0.5 0.5 0.5 1.0]  GraphicAmbientColor=[0.15 0.15 0.15 1.0]  GraphicEmissiveColor=[0.0 0.0 0.0 1.0]  GraphicShininess=75  DoExposeReferenceFrame=on  SerializedFrames=<Frames/>
  pipes : sm_lib/Body Elements/File Solid  ExtGeomFileName=pipes.stl  UnitType=Custom  ExtGeomFileUnits=mm  StepReaderType=HEX  ExportConvexHullGeometry=off  InertiaType=Custom  BasedOnType=DensityFromFile  Density=1000  DensityUnits=kg/m^3  Mass=1  MassUnits=kg  CenterOfMass=[0 0 0]  CenterOfMassUnits=m  MomentsOfInertia=[1 1 1]  MomentsOfInertiaUnits=kg*m^2  ProductsOfInertia=[0 0 0]  ProductsOfInertiaUnits=kg*m^2  GraphicType=FromGeometry  MarkerShape=Sphere  MarkerSize=10  GraphicVisPropType=FromFileVisualProperties  GraphicDiffuseColor=[1.0 1.0 1.0]  GraphicOpacity=1.0  GraphicSpecularColor=[0.5 0.5 0.5 1.0]  GraphicAmbientColor=[0.15 0.15 0.15 1.0]  GraphicEmissiveColor=[0.0 0.0 0.0 1.0]  GraphicShininess=75  DoExposeReferenceFrame=on  SerializedFrames=<Frames/>
  reservoir : sm_lib/Body Elements/File Solid  ExtGeomFileName=reservoir.stl  UnitType=Custom  ExtGeomFileUnits=mm  StepReaderType=HEX  ExportConvexHullGeometry=off  InertiaType=Custom  BasedOnType=DensityFromFile  Density=1000  DensityUnits=kg/m^3  Mass=1  MassUnits=kg  CenterOfMass=[0 0 0]  CenterOfMassUnits=m  MomentsOfInertia=[1 1 1]  MomentsOfInertiaUnits=kg*m^2  ProductsOfInertia=[0 0 0]  ProductsOfInertiaUnits=kg*m^2  GraphicType=FromGeometry  MarkerShape=Sphere  MarkerSize=10  GraphicVisPropType=SimpleVisualProperties  GraphicDiffuseColor=[0.4 0.8 1.0]  GraphicOpacity=0.75  GraphicSpecularColor=[0.5 0.5 0.5 1.0]  GraphicAmbientColor=[0.15 0.15 0.15 1.0]  GraphicEmissiveColor=[0.0 0.0 0.0 1.0]  GraphicShininess=75  DoExposeReferenceFrame=on  SerializedFrames=<Frames/>
  obase : PMIOPort  Side=Left
  connections:
  base/RConn1 -- FV/RConn1 -- Rigid Transform5/LConn1 -- LV/RConn1 -- reservoir/RConn1 -- obase/RConn1 -- pipes/RConn1
  Rigid Transform5/RConn1 -- ac_pump/RConn1

== matlab function labA23/Model/Tank 1/MATLAB Function1 ==
  data: h1 input; dp output; rho parameter; g parameter; h_v1 parameter; h1_min parameter
function dp = delta_p_v1(h1, rho, g, h_v1, h1_min)
%#codegen
if h1 > h1_min
    dp = rho*g*(h1 + h_v1);
else
    dp = 0;
end

== matlab function labA23/Model/Tank 2/MATLAB Function ==
  data: h2 input; dp output; rho parameter; g parameter; h_v2 parameter; h2_min parameter
function dp = delta_p_v2(h2, rho, g, h_v2, h2_min)
%#codegen
if h2 > h2_min
    dp = rho*g*(h2 + h_v2);
else
    dp = 0;
end
